simulink model "AnalyticalModel"  (R2019a)
settings: Solver=VariableStepAuto  StartTime=0.0  StopTime=10.0  RelTol=1e-3
values from neighbouring files (symbols this model uses):
  M1_PhaseA_Ls = 3.3e-3    (= 0.0033)    [AnalyticalParameters.m]
  M1_PhaseB_Ls = 3.3e-3    (= 0.0033)    [AnalyticalParameters.m]
  M1_PhaseC_Ls = 3.3e-3    (= 0.0033)    [AnalyticalParameters.m]
  SamplingTime = 1e-6    (= 1e-06)    [AnalyticalParameters.m]
undefined symbols (not defined in the file or in its folder): Rload
libraries: powerlib x13
settings Model: Creator=admin  LastModifiedBy=admin

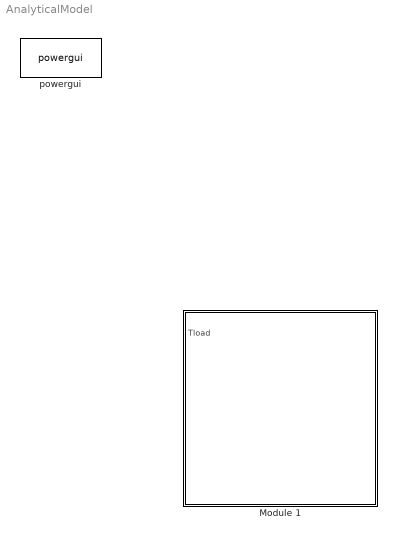
== system AnalyticalModel ==
  Module 1 : Subsystem
  powergui : powerlib/powergui  Priority=1  SimulationMode=Discrete  SampleTime=SamplingTime  frequency=60  Iterations=50  frequencyindice=0  Pbase=100e6  ErrMax=1e-4  UnitsV=kV  UnitsW=MW  buscounter=0  FunctionMessages=off  echomessages=off  EnableUseOfTLC=off  CurrentSourceSwitches=off  DisableSnubberDevices=off  DisableRonSwitches=off  DisableVfSwitches=off  DisplayEquations=off  AutomaticDiscreteSolvers=off  SolverType=Tustin/Backward Euler (TBE)  Interpol=off  ExternalGateDelay=off  methode=off  Ts=100  x0status=blocks  SPID=on  SwTol=0  HookPort=off  NonlinearTolerance=0  nMaxIteration=15  ContinueOnMaxIteration=off  RestoreLinks=warning  ResistiveCurrentMeasurement=off  Frange=[0:2:500]  Ylog=off  Xlog=on  ShowGrid=off  save=off  variable=ZData  structure=0  ZoomFFT=off  StartTime=0.0  cycles=1  DisplayStyle=1  fundamental=60  FreqAxis=off  MaxFrequency=1000  frequencyindicesteady=1  RmsSteady=1  display=off
      settings: SourceProductName=Simscape Electrical

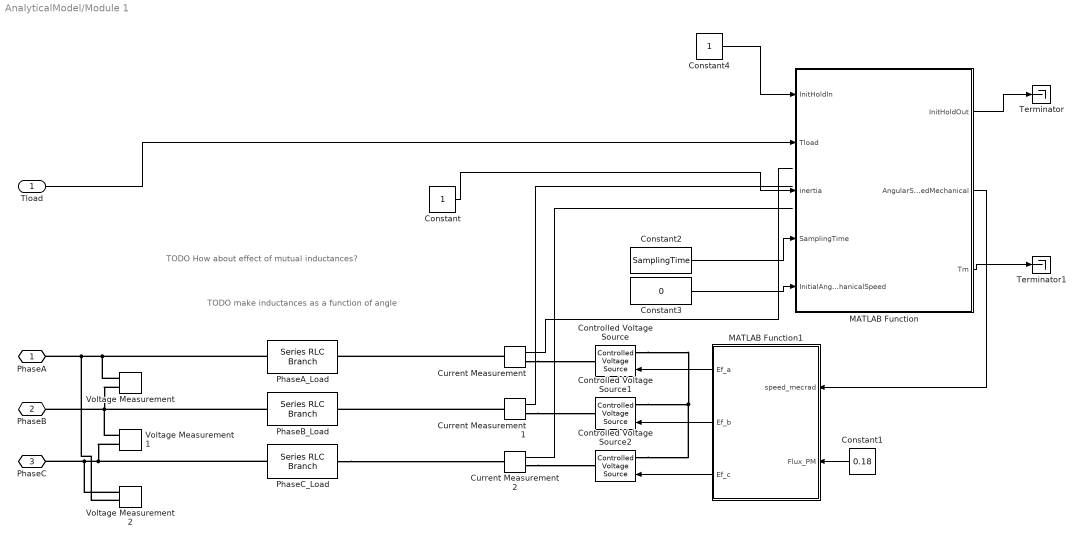
== system AnalyticalModel/Module 1 ==
  note: TODO How about effect of mutual inductances?
  note: TODO make inductances as a function of angle
  Tload : Inport
  Constant : Constant
  Constant1 : Constant  Value=0.18
  Constant2 : Constant  Value=SamplingTime
  Constant3 : Constant  Value=0
  Constant4 : Constant
  Controlled Voltage Source : powerlib/Electrical Sources/Controlled Voltage Source  Initialize=off  Source_Type=AC  Amplitude=0  Phase=0  Frequency=0  Measurements=None
      settings: SourceProductName=Simscape Electrical
  Controlled Voltage Source1 : powerlib/Electrical Sources/Controlled Voltage Source  Initialize=off  Source_Type=AC  Amplitude=0  Phase=0  Frequency=0  Measurements=None
      settings: SourceProductName=Simscape Electrical
  Controlled Voltage Source2 : powerlib/Electrical Sources/Controlled Voltage Source  Initialize=off  Source_Type=AC  Amplitude=0  Phase=0  Frequency=0  Measurements=None
      settings: SourceProductName=Simscape Electrical
  Current Measurement : powerlib/Measurements/Current Measurement  PhasorSimulation=off  OutputType=Complex  PSBequivalent=0
      settings: SourceProductName=Simscape Electrical
  Current Measurement1 : powerlib/Measurements/Current Measurement  PhasorSimulation=off  OutputType=Complex  PSBequivalent=0
      settings: SourceProductName=Simscape Electrical
  Current Measurement2 : powerlib/Measurements/Current Measurement  PhasorSimulation=off  OutputType=Complex  PSBequivalent=0
      settings: SourceProductName=Simscape Electrical
  MATLAB Function : MATLAB Function  TreatAsAtomicUnit=on
  MATLAB Function1 : MATLAB Function  TreatAsAtomicUnit=on
  PhaseA_Load : powerlib/Elements/Series RLC Branch  LConnTagsString=__new0  RConnTagsString=__new0  BranchType=L  Resistance=Rload  Inductance=M1_PhaseA_Ls  SetiL0=off  InitialCurrent=0  Capacitance=1e-6  Setx0=off  InitialVoltage=0  Measurements=None
      settings: SourceProductName=Simscape Electrical
  PhaseB_Load : powerlib/Elements/Series RLC Branch  LConnTagsString=__new0  RConnTagsString=__new0  BranchType=L  Resistance=Rload  Inductance=M1_PhaseB_Ls  SetiL0=off  InitialCurrent=0  Capacitance=1e-6  Setx0=off  InitialVoltage=0  Measurements=None
      settings: SourceProductName=Simscape Electrical
  PhaseC_Load : powerlib/Elements/Series RLC Branch  LConnTagsString=__new0  RConnTagsString=__new0  BranchType=L  Resistance=Rload  Inductance=M1_PhaseC_Ls  SetiL0=off  InitialCurrent=0  Capacitance=1e-6  Setx0=off  InitialVoltage=0  Measurements=None
      settings: SourceProductName=Simscape Electrical
  Terminator : Terminator
  Terminator1 : Terminator
  Voltage Measurement : powerlib/Measurements/Voltage Measurement  PhasorSimulation=off  OutputType=Complex  PSBequivalent=0
      settings: SourceProductName=Simscape Electrical
  Voltage Measurement1 : powerlib/Measurements/Voltage Measurement  PhasorSimulation=off  OutputType=Complex  PSBequivalent=0
      settings: SourceProductName=Simscape Electrical
  Voltage Measurement2 : powerlib/Measurements/Voltage Measurement  PhasorSimulation=off  OutputType=Complex  PSBequivalent=0
      settings: SourceProductName=Simscape Electrical
  PhaseA : PMIOPort  Side=Left
  PhaseB : PMIOPort  Port=2  Side=Left
  PhaseC : PMIOPort  Port=3  Side=Left
  wires:
  Tload/1 -> MATLAB Function/2(Tload)
  Current Measurement/1 -> ?
  Current Measurement1/1 -> ?
  Current Measurement2/1 -> ?
  MATLAB Function1/2(Ef_b) -> Controlled Voltage Source1/1
  MATLAB Function1/1(Ef_a) -> Controlled Voltage Source/1
  MATLAB Function1/3(Ef_c) -> Controlled Voltage Source2/1
  MATLAB Function/2(AngularSpeedMechanical) -> MATLAB Function1/1(speed_mecrad)
  Constant/1 -> MATLAB Function/3(inertia)
  Constant1/1 -> MATLAB Function1/2(Flux_PM)
  Constant2/1 -> MATLAB Function/4(SamplingTime)
  Constant3/1 -> MATLAB Function/5(InitialAngularMechanicalSpeed)
  Constant4/1 -> MATLAB Function/1(InitHoldIn)
  MATLAB Function/1(InitHoldOut) -> Terminator/1
  MATLAB Function/3(Tm) -> Terminator1/1
  connections:
  Controlled Voltage Source1/LConn1 -- Controlled Voltage Source2/LConn1 -- Controlled Voltage Source/LConn1
  PhaseB_Load/LConn1 -- Voltage Measurement1/LConn1 -- Voltage Measurement/LConn2 -- PhaseB/RConn1
  PhaseA_Load/LConn1 -- Voltage Measurement/LConn1 -- Voltage Measurement2/LConn2 -- PhaseA/RConn1
  PhaseC_Load/LConn1 -- Voltage Measurement1/LConn2 -- Voltage Measurement2/LConn1 -- PhaseC/RConn1
  Current Measurement/LConn1 -- PhaseA_Load/RConn1
  Current Measurement/RConn1 -- Controlled Voltage Source/RConn1
  Current Measurement1/LConn1 -- PhaseB_Load/RConn1
  Current Measurement1/RConn1 -- Controlled Voltage Source1/RConn1
  PhaseC_Load/RConn1 -- Current Measurement2/LConn1
  Current Measurement2/RConn1 -- Controlled Voltage Source2/RConn1

== matlab function AnalyticalModel/Module 1/MATLAB Function1 ==
  data: speed_mecrad input; Ef_a output; Ef_b output; Ef_c output; Flux_PM input
function [Ef_a, Ef_b, Ef_c] = fcn(speed_mecrad, Flux_PM)
Ef_a=1;
Ef_b=1;
Ef_c=1;
y = speed_mecrad;

== matlab function AnalyticalModel/Module 1/MATLAB Function ==
  data: InitHoldIn input; InitHoldOut output; Tload input; AngularSpeedMechanical output; inertia input; Tm output; SamplingTime input; InitialAngularMechanicalSpeed input
function [InitHoldOut,AngularSpeedMechanical, Tm]   = fcn(InitHoldIn,Tload,inertia,SamplingTime,InitialAngularMechanicalSpeed)
persistent pAngularSpeedMechanical
persistent pPrevAngularSpeedMechanical
if isempty(pAngularSpeedMechanical)
    pAngularSpeedMechanical = InitialAngularMechanicalSpeed;
    pPrevAngularSpeedMechanical = InitialAngularMechanicalSpeed;
    AngularAcceleration = (pAngularSpeedMechanical-pPrevAngularSpeedMechanical);
    AngularSpeedMechanical = pAngularSpeedMechanical;
else
    AngularAcceleration = (pAngularSpeedMechanical-pPrevAngularSpeedMechanical);
    pAngularSpeedMechanical = pAngularSpeedMechanical+AngularAcceleration*SamplingTime;
    AngularSpeedMechanical = pAngularSpeedMechanical;
end

InitHoldOut=0;
    Tm = 5;
y = Tload;
